simulink model "sat_model_legacy"  (R2022a)
settings: Solver=ode45  StartTime=0.0  StopTime=10.0  MaxStep=0.01  RelTol=1e-3  EnableMultiTasking=on
libraries: aerolibutil x12, sharedutil x6, sharedtransform x2
settings Model: Creator=richard.adams  LastModifiedBy=Connor Emmons
settings SolverCC: AlgebraicLoopSolver=TrustRegion
settings DataIOCC: LimitDataPoints=on  SaveFormat=Array  SignalLoggingSaveFormat=ModelDataLogs  ReturnWorkspaceOutputs=off
settings OptimizationCC: BlockReduction=off  BooleanDataType=off  ExpressionDepthLimit=2147483647  InitFltsAndDblsToZero=on  LifeSpan=inf
settings DebuggingCC: SaveWithParameterizedLinksMsg=none  UnderspecifiedInitializationDetection=Classic  MergeDetectMultiDrivingBlocksExec=none  SignalResolutionControl=TryResolveAllWithWarning  MultiTaskDSMMsg=warning  MultiTaskCondExecSysMsg=none  FcnCallInpInsideContextMsg=warning  UnconnectedInputMsg=warning  UnconnectedOutputMsg=warning  UnconnectedLineMsg=warning  StateNameClashWarn=warning  SFUnexpectedBacktrackingDiag=warning  SFNoUnconditionalDefaultTransitionDiag=warning  SFExecutionAtInitializationDiag=none  ArithmeticOperatorsInVariantConditions=warning
settings HardwareCC: ProdBitPerPointer=32  ProdBitPerSizeT=32  ProdBitPerPtrDiffT=32  ProdLargestAtomicFloat=None  ProdIntDivRoundTo=Undefined  ProdEndianess=Unspecified  ProdWordSize=32  ProdHWDeviceType=32-bit Generic  TargetUnknown=on
settings ModelReferenceCC: EnableRefExpFcnMdlSchedulingChecks=off  PropagateSignalLabelsOutOfModel=off
settings SFSimCC: SimUseLocalCustomCode=off  CustomCodeUndefinedFunction=UseInterfaceOnly
settings RTWCC: RTWUseLocalCustomCode=off
settings CodeAppCC: StateflowObjectComments=on
settings GRTTargetCC: TargetLangStandard=C89/C90 (ANSI)  CombineOutputUpdateFcns=off  GRTInterface=on
settings ConfigComp: CovMetricSettings=dw  CovSaveCumulativeToWorkspaceVar=on  CovSaveSingleToWorkspaceVar=on  CovExternalEMLEnable=off

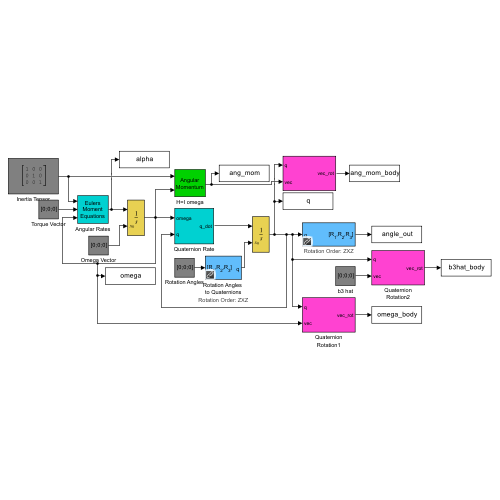
[thumbnail: Simulink's stored preview of the top-level diagram]
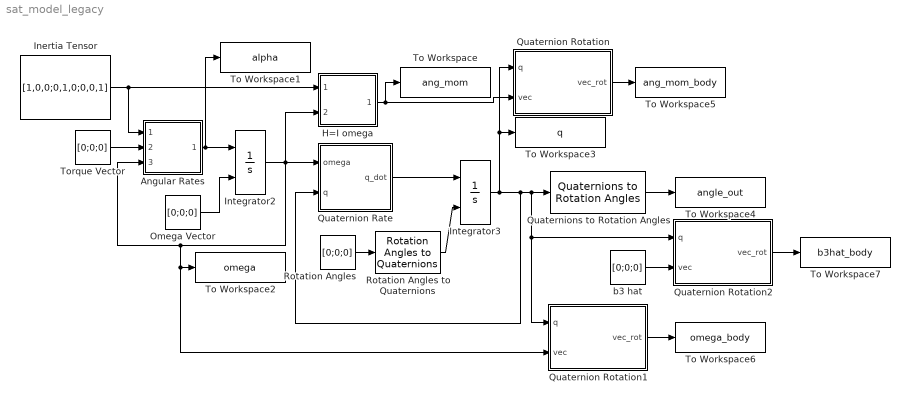
== system sat_model_legacy ==
  Angular Rates : Subsystem  mask(Angular Rate Computation in Body Coordiantes){}
      mask help:
      | Input 1 - 3x3 Inertia Tensor   Output - 3x1 Omega Dot Vector
      | Input 2 - 3x1 Torque Vector
      | Input 3 - 3x1 Omega Vector
      mask Display: disp('Eulers\nMoment\nEquations')
  H=I omega : Subsystem  mask(Angular Momentum Vector Calculation){}
      mask help:
      | Input 1 - 3x3 Inertia Tensor      Output - 3x1 H  Vector
      | Input 2 - 3x1 Omega Vector
      mask Display: disp('Angular\nMomentum')
  Inertia Tensor : Constant  Value=[1,0,0;0,1,0;0,0,1]  VectorParams1D=off
  Integrator2 : Integrator  InitialConditionSource=external  InitialCondition=[0;0;0]
  Integrator3 : Integrator  InitialConditionSource=external  InitialCondition=[0;0;0]
  Omega Vector : Constant  Value=[0;0;0]
  Quaternion Rotation : Subsystem
  Quaternion Rotation1 : Subsystem
  Quaternion Rotation2 : Subsystem
  Quaternion Rate : Subsystem
  Quaternions to Rotation Angles : sharedtransform/Quaternions to Rotation Angles  rotationOrder=ZXZ  aMode=aMode
  Rotation Angles : Constant  Value=[0;0;0]
  Rotation Angles to Quaternions : sharedtransform/Rotation Angles to Quaternions  rotationOrder=ZXZ  aMode=aMode
  To Workspace : ToWorkspace  VariableName=ang_mom  SampleTime=-1
  To Workspace1 : ToWorkspace  VariableName=alpha  SampleTime=-1
  To Workspace2 : ToWorkspace  VariableName=omega  SampleTime=-1
  To Workspace3 : ToWorkspace  VariableName=q  SaveFormat=Timeseries  SampleTime=-1
  To Workspace4 : ToWorkspace  VariableName=angle_out  SaveFormat=Timeseries  SampleTime=-1
  To Workspace5 : ToWorkspace  VariableName=ang_mom_body  SampleTime=-1
  To Workspace6 : ToWorkspace  VariableName=omega_body  SampleTime=-1
  To Workspace7 : ToWorkspace  VariableName=b3hat_body  SampleTime=-1
  Torque Vector : Constant  Value=[0;0;0]
  b3 hat : Constant  Value=[0;0;0]
  wires:
  Inertia Tensor/1 -> H=I omega/1(Inertia Tensor), Angular Rates/1(Inertia Tensor)
  Torque Vector/1 -> Angular Rates/2(torque(1) torque(2) torque(3))
  Angular Rates/1(omega dot(1) omega dot(2) omega dot(3)) -> To Workspace1/1, Integrator2/1
  Integrator2/1 -> H=I omega/2(omega(1) omega(2) omega(3)), Quaternion Rotation1/2(vec), To Workspace2/1, Angular Rates/3(omega(1) omega(2) omega(3)), Quaternion Rate/1(omega)
  Omega Vector/1 -> Integrator2/2
  Rotation Angles/1 -> Rotation Angles to Quaternions/1
  Quaternion Rate/1(q_dot) -> Integrator3/1
  Integrator3/1 -> Quaternion Rotation/1(q), To Workspace3/1, Quaternion Rotation2/1(q), Quaternion Rotation1/1(q), Quaternions to Rotation Angles/1, Quaternion Rate/2(q)
  Rotation Angles to Quaternions/1 -> Integrator3/2
  H=I omega/1(H(1) H(2) H(3)) -> Quaternion Rotation/2(vec), To Workspace/1
  Quaternions to Rotation Angles/1 -> To Workspace4/1
  Quaternion Rotation/1(vec_rot) -> To Workspace5/1
  Quaternion Rotation1/1(vec_rot) -> To Workspace6/1
  b3 hat/1 -> Quaternion Rotation2/2(vec)
  Quaternion Rotation2/1(vec_rot) -> To Workspace7/1

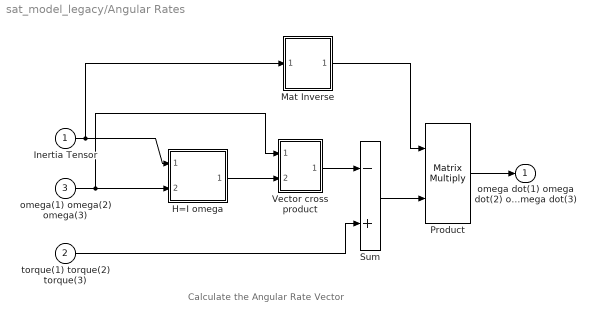
== system sat_model_legacy/Angular Rates ==
  note: Calculate the Angular Rate Vector
  Inertia Tensor : Inport
  torque(1) torque(2) torque(3) : Inport  Port=2
  omega(1) omega(2) omega(3) : Inport  Port=3
  H=I omega : Subsystem  mask(Angular Momentum Vector){}
      mask help: Angular Momentum Vector Calculator
      mask Display: disp('Angular\nMomentum')
  Mat Inverse : Subsystem  mask(Matrix Inverse){}
      mask help: Vector Transformation
      mask Display: disp('Matrix\nInverse')
  Product : Product  Multiplication=Matrix(*)  InputSameDT=on  RndMeth=Zero  SaturateOnIntegerOverflow=on  OutDataTypeStr=Inherit: Same as first input
  Sum : Sum  Inputs=-+  InputSameDT=on  SaturateOnIntegerOverflow=on  OutDataTypeStr=Inherit: Same as first input
  Vector cross product : Subsystem  mask(Cross Product){}
      mask help: Cross Product
      mask Display: disp('Cross\nProduct')
  omega dot(1) omega dot(2) omega dot(3) : Outport  InitialOutput=0
  wires:
  Inertia Tensor/1 -> H=I omega/1(Inertia Tensor), Mat Inverse/1(Input Matrix)
  omega(1) omega(2) omega(3)/1 -> H=I omega/2(omega(1) omega(2) omega(3)), Vector cross product/1(a(1) a(2) a(3))
  torque(1) torque(2) torque(3)/1 -> Sum/2
  H=I omega/1(H(1) H(2) H(3)) -> Vector cross product/2(b(1) b(2) b(3))
  Vector cross product/1(c(1) c(2) c(3)) -> Sum/1
  Sum/1 -> Product/2
  Product/1 -> omega dot(1) omega dot(2) omega dot(3)/1
  Mat Inverse/1(Output Matrix) -> Product/1

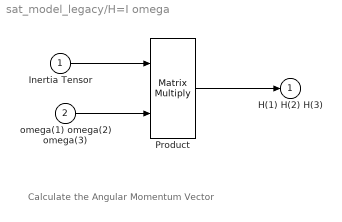
== system sat_model_legacy/H=I omega ==
  note: Calculate the Angular Momentum Vector
  Inertia Tensor : Inport
  omega(1) omega(2) omega(3) : Inport  Port=2
  Product : Product  Multiplication=Matrix(*)  InputSameDT=on  RndMeth=Zero  SaturateOnIntegerOverflow=on  OutDataTypeStr=Inherit: Same as first input
  H(1) H(2) H(3) : Outport  InitialOutput=0
  wires:
  Product/1 -> H(1) H(2) H(3)/1
  Inertia Tensor/1 -> Product/1
  omega(1) omega(2) omega(3)/1 -> Product/2

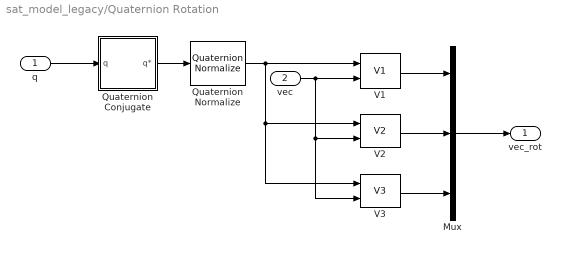
== system sat_model_legacy/Quaternion Rotation ==
  q : Inport  Unit=1
  vec : Inport  Port=2
  Mux : Mux  Inputs=3
  Quaternion Normalize : sharedutil/Quaternion Normalize  aMode=aMode
  Quaternion Conjugate : Subsystem
  V1 : aerolibutil/Quaternion Rotation/V1  SystemSampleTime=-1  VariantActivationTime=update diagram  Latency=0  AutoFrameSizeCalculation=off
  V2 : aerolibutil/Quaternion Rotation/V2  SystemSampleTime=-1  VariantActivationTime=update diagram  Latency=0  AutoFrameSizeCalculation=off
  V3 : aerolibutil/Quaternion Rotation/V3  SystemSampleTime=-1  VariantActivationTime=update diagram  Latency=0  AutoFrameSizeCalculation=off
  vec_rot : Outport  VectorParamsAs1DForOutWhenUnconnected=off
  wires:
  Quaternion Normalize/1 -> V3/1, V2/1, V1/1
  V3/1 -> Mux/3
  Mux/1 -> vec_rot/1
  q/1 -> Quaternion Conjugate/1(q)
  Quaternion Conjugate/1(q*) -> Quaternion Normalize/1
  V2/1 -> Mux/2
  vec/1 -> V3/2, V2/2, V1/2
  V1/1 -> Mux/1

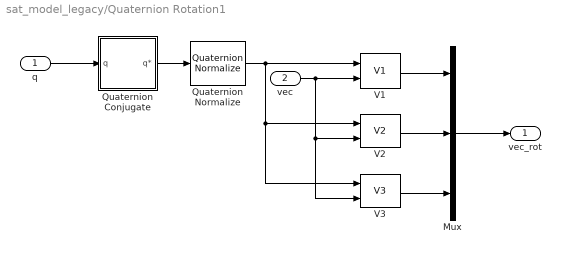
== system sat_model_legacy/Quaternion Rotation1 ==
  q : Inport  Unit=1
  vec : Inport  Port=2
  Mux : Mux  Inputs=3
  Quaternion Normalize : sharedutil/Quaternion Normalize  aMode=aMode
  Quaternion Conjugate : Subsystem
  V1 : aerolibutil/Quaternion Rotation/V1  SystemSampleTime=-1  VariantActivationTime=update diagram  Latency=0  AutoFrameSizeCalculation=off
  V2 : aerolibutil/Quaternion Rotation/V2  SystemSampleTime=-1  VariantActivationTime=update diagram  Latency=0  AutoFrameSizeCalculation=off
  V3 : aerolibutil/Quaternion Rotation/V3  SystemSampleTime=-1  VariantActivationTime=update diagram  Latency=0  AutoFrameSizeCalculation=off
  vec_rot : Outport  VectorParamsAs1DForOutWhenUnconnected=off
  wires:
  Quaternion Normalize/1 -> V3/1, V2/1, V1/1
  V3/1 -> Mux/3
  Mux/1 -> vec_rot/1
  q/1 -> Quaternion Conjugate/1(q)
  Quaternion Conjugate/1(q*) -> Quaternion Normalize/1
  V2/1 -> Mux/2
  vec/1 -> V3/2, V2/2, V1/2
  V1/1 -> Mux/1

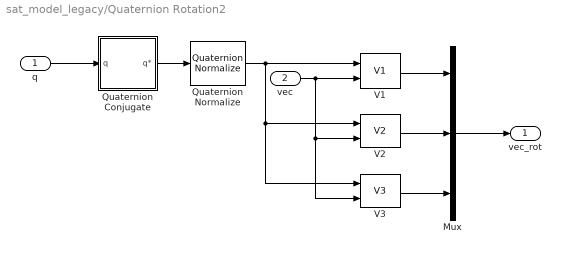
== system sat_model_legacy/Quaternion Rotation2 ==
  q : Inport  Unit=1
  vec : Inport  Port=2
  Mux : Mux  Inputs=3
  Quaternion Normalize : sharedutil/Quaternion Normalize  aMode=aMode
  Quaternion Conjugate : Subsystem
  V1 : aerolibutil/Quaternion Rotation/V1  SystemSampleTime=-1  VariantActivationTime=update diagram  Latency=0  AutoFrameSizeCalculation=off
  V2 : aerolibutil/Quaternion Rotation/V2  SystemSampleTime=-1  VariantActivationTime=update diagram  Latency=0  AutoFrameSizeCalculation=off
  V3 : aerolibutil/Quaternion Rotation/V3  SystemSampleTime=-1  VariantActivationTime=update diagram  Latency=0  AutoFrameSizeCalculation=off
  vec_rot : Outport  VectorParamsAs1DForOutWhenUnconnected=off
  wires:
  Quaternion Normalize/1 -> V3/1, V2/1, V1/1
  V3/1 -> Mux/3
  Mux/1 -> vec_rot/1
  q/1 -> Quaternion Conjugate/1(q)
  Quaternion Conjugate/1(q*) -> Quaternion Normalize/1
  V2/1 -> Mux/2
  vec/1 -> V3/2, V2/2, V1/2
  V1/1 -> Mux/1

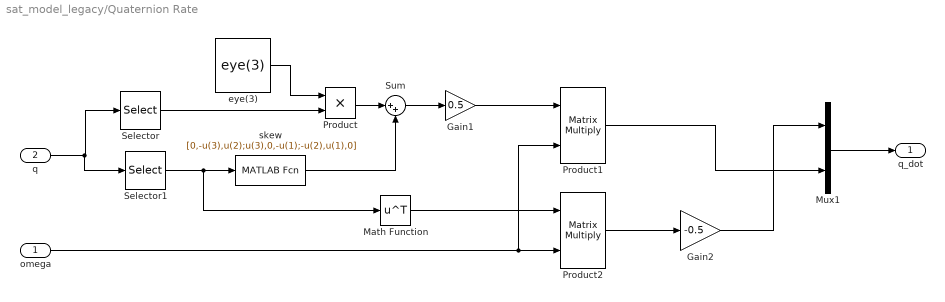
== system sat_model_legacy/Quaternion Rate ==
  omega : Inport
  q : Inport  Port=2
  Gain1 : Gain  Gain=0.5
  Gain2 : Gain  Gain=-0.5
  Math Function : Math  Operator=transpose
  Mux1 : Mux  Inputs=2
  Product : Product
  Product1 : Product  Multiplication=Matrix(*)
  Product2 : Product  Multiplication=Matrix(*)
  Selector : Selector  InputPortWidth=4  IndexOptions=Index vector (dialog)  Indices=[1]  OutputSizes=1
  Selector1 : Selector  InputPortWidth=4  IndexOptions=Index vector (dialog)  Indices=[2 3 4]  OutputSizes=1
  Sum : Sum  Inputs=|++
  eye(3) : Constant  Value=eye(3)
  skew : MATLABFcn  MATLABFcn=[0,-u(3),u(2);u(3),0,-u(1);-u(2),u(1),0]  Output1D=off
  q_dot : Outport
  wires:
  Product2/1 -> Gain2/1
  Product/1 -> Sum/1
  eye(3)/1 -> Product/1
  Math Function/1 -> Product2/1
  Gain2/1 -> Mux1/1
  Product1/1 -> Mux1/2
  Selector1/1 -> Math Function/1, skew/1
  Mux1/1 -> q_dot/1
  skew/1 -> Sum/2
  Gain1/1 -> Product1/1
  Sum/1 -> Gain1/1
  omega/1 -> Product1/2, Product2/2
  q/1 -> Selector1/1, Selector/1
  Selector/1 -> Product/2

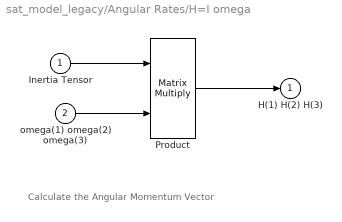
== system sat_model_legacy/Angular Rates/H=I omega ==
  note: Calculate the Angular Momentum Vector
  Inertia Tensor : Inport
  omega(1) omega(2) omega(3) : Inport  Port=2
  Product : Product  Multiplication=Matrix(*)  InputSameDT=on  RndMeth=Zero  SaturateOnIntegerOverflow=on  OutDataTypeStr=Inherit: Same as first input
  H(1) H(2) H(3) : Outport  InitialOutput=0
  wires:
  Product/1 -> H(1) H(2) H(3)/1
  Inertia Tensor/1 -> Product/1
  omega(1) omega(2) omega(3)/1 -> Product/2

== system sat_model_legacy/Angular Rates/Mat Inverse ==
  note: Calculate the Inverse of a Matrix
  Input Matrix : Inport
  MATLAB Fcn : MATLABFcn  MATLABFcn=inv([u(1,1) u(1,2) u(1,3);u(2,1) u(2,2) u(2,3);u(3,1) u(3,2) u(3,3)])  Output1D=off
  Output Matrix : Outport  InitialOutput=0
  wires:
  MATLAB Fcn/1 -> Output Matrix/1
  Input Matrix/1 -> MATLAB Fcn/1

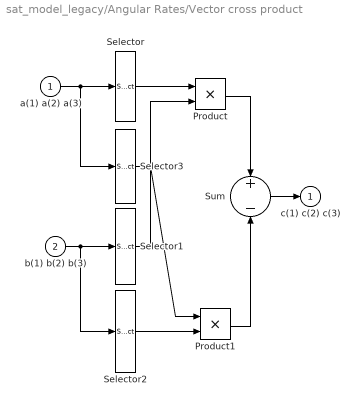
== system sat_model_legacy/Angular Rates/Vector cross product ==
  a(1) a(2) a(3) : Inport
  b(1) b(2) b(3) : Inport  Port=2
  Product : Product  InputSameDT=on  RndMeth=Zero  SaturateOnIntegerOverflow=on  OutDataTypeStr=Inherit: Same as first input
  Product1 : Product  InputSameDT=on  RndMeth=Zero  SaturateOnIntegerOverflow=on  OutDataTypeStr=Inherit: Same as first input
  Selector : Selector  InputPortWidth=3  IndexOptions=Index vector (dialog)  Indices=[2 3 1]  OutputSizes=1
  Selector1 : Selector  InputPortWidth=3  IndexOptions=Index vector (dialog)  Indices=[3 1 2]  OutputSizes=1
  Selector2 : Selector  InputPortWidth=3  IndexOptions=Index vector (dialog)  Indices=[2 3 1]  OutputSizes=1
  Selector3 : Selector  InputPortWidth=3  IndexOptions=Index vector (dialog)  Indices=[3 1 2]  OutputSizes=1
  Sum : Sum  Inputs=+|-  InputSameDT=on  SaturateOnIntegerOverflow=on  OutDataTypeStr=Inherit: Same as first input
  c(1) c(2) c(3) : Outport  InitialOutput=0
  wires:
  Sum/1 -> c(1) c(2) c(3)/1
  b(1) b(2) b(3)/1 -> Selector1/1, Selector2/1
  Selector/1 -> Product/1
  a(1) a(2) a(3)/1 -> Selector/1, Selector3/1
  Product/1 -> Sum/1
  Selector1/1 -> Product/2
  Product1/1 -> Sum/2
  Selector2/1 -> Product1/2
  Selector3/1 -> Product1/1

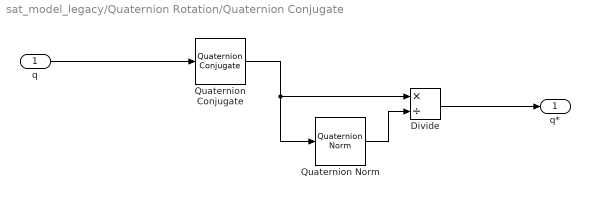
== system sat_model_legacy/Quaternion Rotation/Quaternion Conjugate ==
  q : Inport
  Divide : Product  Inputs=*/
  Quaternion Conjugate : aerolibutil/Quaternion Conjugate
  Quaternion Norm : sharedutil/Quaternion Norm  aMode=aMode
  q* : Outport
  wires:
  q/1 -> Quaternion Conjugate/1
  Divide/1 -> q*/1
  Quaternion Conjugate/1 -> Quaternion Norm/1, Divide/1
  Quaternion Norm/1 -> Divide/2

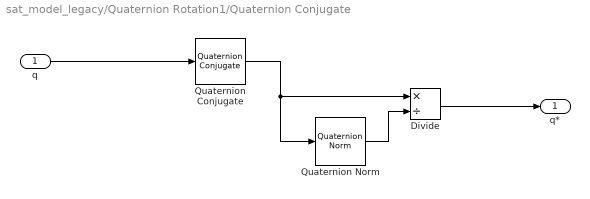
== system sat_model_legacy/Quaternion Rotation1/Quaternion Conjugate ==
  q : Inport
  Divide : Product  Inputs=*/
  Quaternion Conjugate : aerolibutil/Quaternion Conjugate
  Quaternion Norm : sharedutil/Quaternion Norm  aMode=aMode
  q* : Outport
  wires:
  q/1 -> Quaternion Conjugate/1
  Divide/1 -> q*/1
  Quaternion Conjugate/1 -> Quaternion Norm/1, Divide/1
  Quaternion Norm/1 -> Divide/2

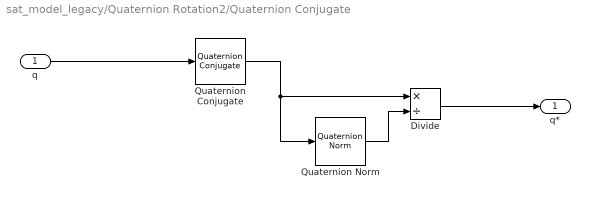
== system sat_model_legacy/Quaternion Rotation2/Quaternion Conjugate ==
  q : Inport
  Divide : Product  Inputs=*/
  Quaternion Conjugate : aerolibutil/Quaternion Conjugate
  Quaternion Norm : sharedutil/Quaternion Norm  aMode=aMode
  q* : Outport
  wires:
  q/1 -> Quaternion Conjugate/1
  Divide/1 -> q*/1
  Quaternion Conjugate/1 -> Quaternion Norm/1, Divide/1
  Quaternion Norm/1 -> Divide/2
